simulink model "modelo_motor_espaco_estados"  (R2020b)
settings: Solver=VariableStepAuto  StartTime=0.0  StopTime=10  RelTol=1e-3
values from neighbouring files (symbols this model uses):
  A = [-676.470588235  -206.018789225; 26.2510368664  -1.40591397849]    [motor.mat]
  B = [294.117647059 0]    [motor.mat]
  C = [0 1]    [motor.mat]
  finalvalue = 5    [motor.mat]
  initialvalue = 0    [motor.mat]
  Kt = 0.0215571428571    [motor.mat]
  steptime = 1    [motor.mat]
libraries: simulink x4
settings Model: Creator=gusta  LastModifiedBy=lucas
settings DebuggingCC: SFMachineParentedDataDiag=error

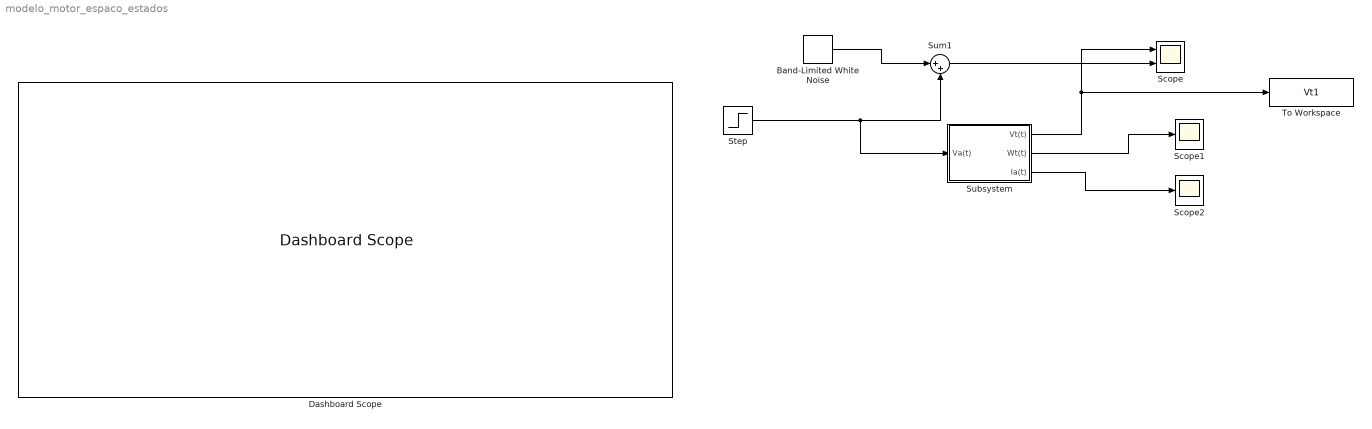
== system modelo_motor_espaco_estados ==
  Band-Limited White Noise : simulink/Sources/Band-Limited White Noise  Cov=[0.000001]  Ts=0.001  seed=[23341]
  Dashboard Scope : DashboardScope  Ymin=-20  Ymax=20
  Scope : Scope  NumInputPorts=2
  Scope1 : Scope
  Scope2 : Scope
  Step : Step  Time=steptime  Before=initialvalue  After=finalvalue  SampleTime=0
  Subsystem : Subsystem
  Sum1 : Sum  Inputs=|++
  To Workspace : ToWorkspace  VariableName=Vt1  SaveFormat=Structure With Time  SampleTime=-1
  wires:
  Subsystem/1(Vt(t)) -> To Workspace/1, Scope/1
  Subsystem/2(Wt(t)) -> Scope1/1
  Subsystem/3(Ia(t)) -> Scope2/1
  Sum1/1 -> Scope/2
  Band-Limited White Noise/1 -> Sum1/1
  Step/1 -> Subsystem/1(Va(t)), Sum1/2

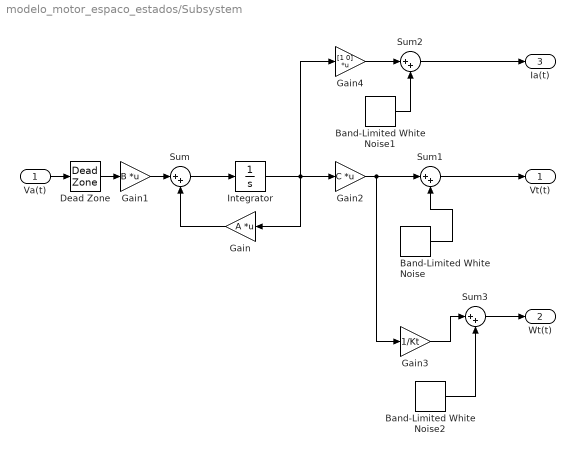
== system modelo_motor_espaco_estados/Subsystem ==
  Va(t) : Inport
  Band-Limited White Noise : simulink/Sources/Band-Limited White Noise  Cov=[0.000005]  Ts=0.001  seed=[23341]
  Band-Limited White Noise1 : simulink/Sources/Band-Limited White Noise  Cov=[0.00000001]  Ts=0.001  seed=[23341]
  Band-Limited White Noise2 : simulink/Sources/Band-Limited White Noise  Cov=[0.0007]  Ts=0.001  seed=[23341]
  Dead Zone : DeadZone  LowerValue=-3.2  UpperValue=3.2  SaturateOnIntegerOverflow=on
  Gain : Gain  Gain=A  Multiplication=Matrix(K*u)
  Gain1 : Gain  Gain=B  Multiplication=Matrix(K*u)
  Gain2 : Gain  Gain=C  Multiplication=Matrix(K*u)
  Gain3 : Gain  Gain=1/Kt
  Gain4 : Gain  Gain=[1 0]  Multiplication=Matrix(K*u)
  Integrator : Integrator
  Sum{,1..3} (4 alike) : Sum  Inputs=|++
  Vt(t) : Outport
  Wt(t) : Outport  Port=2
  Ia(t) : Outport  Port=3
  wires:
  Sum/1 -> Integrator/1
  Integrator/1 -> Gain4/1, Gain2/1, Gain/1
  Gain2/1 -> Sum1/1, Gain3/1
  Gain1/1 -> Sum/1
  Gain/1 -> Sum/2
  Va(t)/1 -> Dead Zone/1
  Dead Zone/1 -> Gain1/1
  Sum1/1 -> Vt(t)/1
  Band-Limited White Noise/1 -> Sum1/2
  Sum2/1 -> Ia(t)/1
  Gain4/1 -> Sum2/1
  Sum3/1 -> Wt(t)/1
  Band-Limited White Noise1/1 -> Sum2/2
  Band-Limited White Noise2/1 -> Sum3/2
  Gain3/1 -> Sum3/1
